simulink model "AVAS_Simulation"  (R2024b)
settings: Solver=ode45  StartTime=0.0  StopTime=20.00  FixedStep=0.001  RelTol=1e-3
libraries: dspsnks4 x1, simulink x1, SignalEditorBlockLib x1
settings Model: PacingRate=0.400000  Creator=KIIT0001  LastModifiedBy=KIIT0001

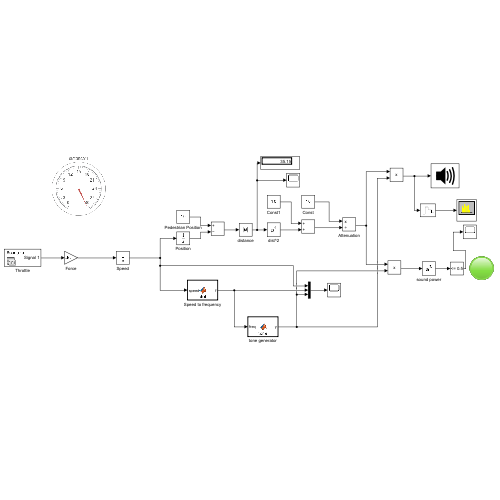
[thumbnail: Simulink's stored preview of the top-level diagram]
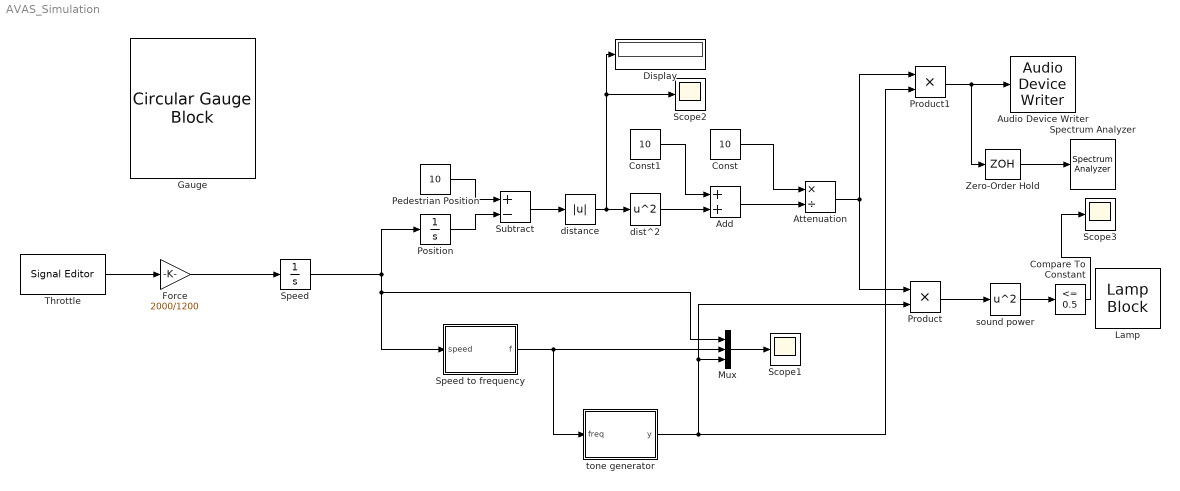
== system AVAS_Simulation ==
  Add : Sum
  Attenuation : Product  Inputs=*/
  Audio Device Writer : dspsnks4/Audio Device Writer  Driver=DirectSound  Device=Default  InheritSampleRate=off  SampleRate=44100  BitDepth=16-bit integer  BufferSize=4096  NumBuffers=10  DefaultOutputChannelMapping=on  OutputChannelMapping=1:2  OutputNumUnderrunSamples=off  DriverIdx=1  DeviceWarnFlag=''
  Compare To Constant : simulink/Logic and Bit Operations/Compare To Constant  relop=<=  const=0.5  OutDataTypeStr=boolean
  Const : Constant  Value=10
  Const1 : Constant  Value=10
  Display : Display
  Force : Gain  Gain=2000/1200
  Gauge : CircularGaugeBlock  ScaleMax=30
  Lamp : LampBlock  LabelPosition=Hide
  Mux : Mux  Inputs=3
  Pedestrian Position : Constant  Value=10
  Position : Integrator
  Product : Product
  Product1 : Product
  Scope1 : Scope
  Scope2 : Scope
  Scope3 : Scope
  Spectrum Analyzer : SpectrumAnalyzer  WindowPosition=[121.000000,-82.000000,800.000000,500.000000,]  ScopeFrameLocation=window  SampleRate=44.1e3  PlotAsTwoSidedSpectrum=off  FrequencyScale=Log  WindowInvariantSamplesPerUpdate=on  FrequencySpan=Start and stop frequencies  StartFrequency=20  StopFrequency=20e3  YLimits=[-148.41731959,7.5332664]
  Speed : Integrator
  Speed to frequency : MATLAB Function  TreatAsAtomicUnit=on
  Subtract : Sum  Inputs=+-
  Throttle : SignalEditorBlockLib/Signal Editor  FileName=throttle.mat  ActiveScenario=Scenario  ActiveSignal=Signal 1  IsBus=off  OutputBusObjectStr=Bus: BusObject  SampleTime=0  Interpolate=off  ZeroCross=off  OutputAfterFinalValue=Setting to zero  Unit=inherit  PreserveSignalName=on  ApplySigPropsToAllScenarios=on  ApplySigPropsToAllSignals=off
  Zero-Order Hold : ZeroOrderHold  SampleTime=1/44100
  dist^2 : Math  Operator=square
  distance : Abs  SaturateOnIntegerOverflow=off
  sound power : Math  Operator=square
  tone generator : MATLAB Function  TreatAsAtomicUnit=on
  wires:
  Throttle/1 -> Force/1
  Force/1 -> Speed/1
  Speed/1 -> Mux/1, Speed to frequency/1(speed), Position/1
  Speed to frequency/1(f) -> Mux/2, tone generator/1(freq)
  Mux/1 -> Scope1/1
  tone generator/1(y) -> Product1/2, Product/2, Mux/3
  Pedestrian Position/1 -> Subtract/1
  Position/1 -> Subtract/2
  Subtract/1 -> distance/1
  distance/1 -> Scope2/1, Display/1, dist^2/1
  Const1/1 -> Add/1
  dist^2/1 -> Add/2
  Const/1 -> Attenuation/1
  Add/1 -> Attenuation/2
  Attenuation/1 -> Product1/1, Product/1
  Product/1 -> sound power/1
  sound power/1 -> Compare To Constant/1
  Compare To Constant/1 -> Scope3/1
  Product1/1 -> Zero-Order Hold/1, Audio Device Writer/1
  Zero-Order Hold/1 -> Spectrum Analyzer/1

== matlab function AVAS_Simulation/Speed to frequency ==
  data: speed input; f output
function f = stof(speed)

base = 200;      
k = 25;          

f = base + k*speed;

end

== matlab function AVAS_Simulation/tone generator ==
  settings: updateMethod=DISCRETE
  data: freq input; y output
function y = tone(freq)

persistent t
if isempty(t)
    t = 0;
end

fs = 44100;
dt = 1/fs;

y = sin(2*pi*freq*t) ...
  + 0.5*sin(2*pi*2*freq*t) ...
  + 0.25*sin(2*pi*3*freq*t);

t = t + dt;

end
